simulink model "G2VHDV4"  (R2018b)
settings: Solver=VariableStepAuto  StartTime=0.0  StopTime=1  RelTol=1e-3
undefined symbols (not defined in the file): Ion, Lithium
libraries: powerlib x20, electricdrivelib x1, powerlib_meascontrol x1
settings Model: Creator=user  LastModifiedBy=utkar

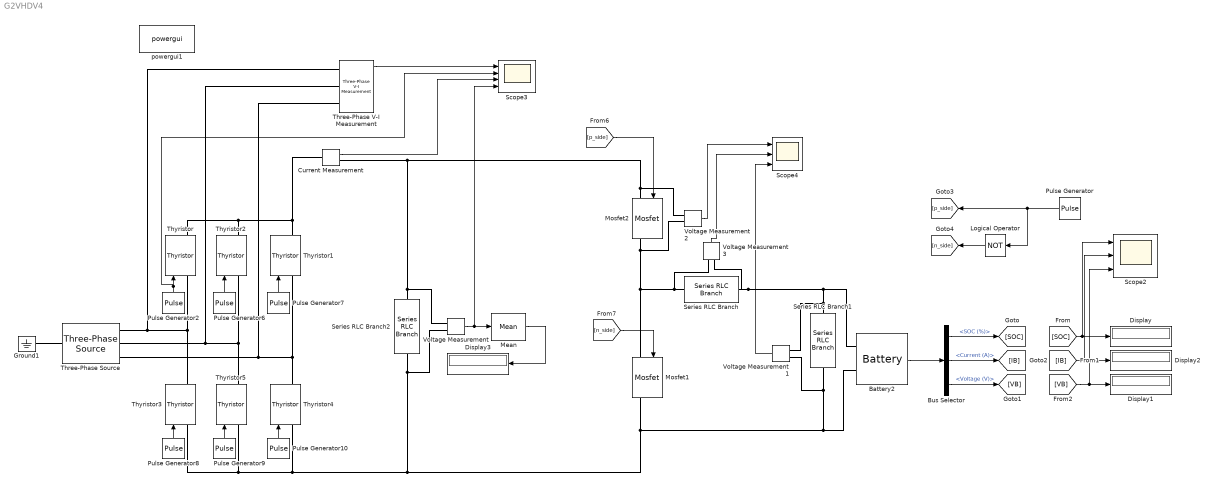
== system G2VHDV4 ==
  Battery2 : electricdrivelib/Extra Sources/Battery  BatType=Lithium-Ion  ShowTempParam=off  ThermalPreset=no  ShowAgeParam=off  NomV=24  NomQ=10  SOC=50  Batt_Tr=1e-4  PresetModel=on  MaxQ=10  MinV=18  FullV=27.9357  Dis_rate=4.3478  R=0.024  Normal_OP=9.0435  expZone="[25.9293     0.491304]"  current=[6.5 13 32.5]  Units=Time  Tci=20  NomT=20  T2=-30  MaxQ2=4.8  FullV2=7.1  Normal_OP2=5.655  expZone2="[6.58           1]"  Rca=0.6  ti=2000  Dp=0  Neq0=0  Tsim=1e6  Ta1=25  Qeol=5.4*0.9  Reol=0.013333*1.2  Char_age=[2.3478, 3]  Dis_age=[2.3478, 10]  N1=1500  N2=10500  N3=1000  N4=1400  Ta2=45  N5=950
  Bus Selector : BusSelector  OutputSignals=SOC (%),Current (A),Voltage (V)
  Current Measurement : powerlib/Measurements/Current Measurement  PhasorSimulation=off  OutputType=Complex  PSBequivalent=0
  Display{,1..3} (4 alike) : Display
  Ground1 : powerlib/Elements/Ground  LConnTagsString=a
  Logical Operator : Logic  Operator=NOT  AllPortsSameDT=off  OutDataTypeStr=boolean
  Mean : powerlib_meascontrol/Measurements/Mean  Freq=50  Vinit=0  Ts=0
  Mosfet1 : powerlib/Power Electronics/Mosfet  Ron=0.1  Lon=0  Rd=0.01  Vfd=0  IC=0  Rs=1e5  Cs=inf  Measurements=on
  Mosfet2 : powerlib/Power Electronics/Mosfet  Ron=0.1  Lon=0  Rd=0.01  Vfd=0  IC=0  Rs=1e5  Cs=inf  Measurements=on
  Pulse Generator : DiscretePulseGenerator  PulseType=Time based  Period=1e-4  PulseWidth=70
  Pulse Generator10 : DiscretePulseGenerator  PulseType=Time based  Period=0.02  PulseWidth=10  PhaseDelay=(1.667e-3)*3+(5.388e-3)
  Pulse Generator2 : DiscretePulseGenerator  PulseType=Time based  Period=0.02  PulseWidth=10  PhaseDelay=(1.667e-3)+(5.388e-3)
  Pulse Generator6 : DiscretePulseGenerator  PulseType=Time based  Period=0.02  PulseWidth=10  PhaseDelay=(1.667e-3)*5+(5.388e-3)
  Pulse Generator7 : DiscretePulseGenerator  PulseType=Time based  Period=0.02  PulseWidth=10  PhaseDelay=(1.667e-3)*9+(5.388e-3)
  Pulse Generator8 : DiscretePulseGenerator  PulseType=Time based  Period=0.02  PulseWidth=10  PhaseDelay=(1.667e-3)*7+(5.388e-3)
  Pulse Generator9 : DiscretePulseGenerator  PulseType=Time based  Period=0.02  PulseWidth=10  PhaseDelay=(1.667e-3)*11+(5.388e-3)
  Scope2 : Scope  NumInputPorts=3
  Scope3 : Scope  NumInputPorts=4
  Scope4 : Scope  NumInputPorts=3
  Series RLC Branch : powerlib/Elements/Series RLC Branch  LConnTagsString=__new0  RConnTagsString=__new0  BranchType=RL  Resistance=0.1  Inductance=1e-3  SetiL0=off  InitialCurrent=0  Capacitance=1e-6  Setx0=off  InitialVoltage=0  Measurements=None
  Series RLC Branch1 : powerlib/Elements/Series RLC Branch  LConnTagsString=__new0  RConnTagsString=__new0  BranchType=RC  Resistance=0.001  Inductance=1e-3  SetiL0=off  InitialCurrent=0  Capacitance=1000e-6  Setx0=off  InitialVoltage=0  Measurements=None
  Series RLC Branch2 : powerlib/Elements/Series RLC Branch  LConnTagsString=__new0  RConnTagsString=__new0  BranchType=R  Resistance=10  Inductance=30e-3  SetiL0=off  InitialCurrent=0  Capacitance=1e-6  Setx0=off  InitialVoltage=0  Measurements=None
  Three-Phase V-I Measurement : powerlib/Measurements/Three-Phase V-I Measurement  VoltageMeasurement=phase-to-ground  SetLabelV=off  LabelV=Vabc  Vpu=off  VpuLL=off  CurrentMeasurement=no  SetLabelI=off  LabelI=Iabc  Ipu=off  Pbase=100e6  Vbase=500e3  OutputType=Complex  PhasorSimulation=off  PSBequivalent=0
  Three-Phase Source : powerlib/Electrical Sources/Three-Phase Source  InternalConnection=Yn  VoltagePhases=off  Voltage=398  PhaseAngle=0  Voltage_phases=[25e3 25e3 25e3]/sqrt(3)  PhaseAngles_phases=[0 -120 +120]  Frequency=50  NonIdealSource=on  SpecifyImpedance=off  Resistance=0  Inductance=0  ShortCircuitLevel=100e6  BaseVoltage=0  XRratio=7  BusType=swing  Pref=10e3  Qref=0  Prefabc=[10e3, 10e3, 10e3]  Qrefabc=[0, 0, 0]  Qmin=-inf  Qmax=inf
  Thyristor{,1..5} (6 alike) : powerlib/Power Electronics/Thyristor  Ron=0  Lon=0  Vf=0  IC=0  Rs=0  Cs=0  Measurements=on
  Voltage Measurement{,1..3} (4 alike) : powerlib/Measurements/Voltage Measurement  PhasorSimulation=off  OutputType=Complex  PSBequivalent=0
  powergui1 : powerlib/powergui  Priority=1  SimulationMode=Continuous  SampleTime=50e-6  frequency=60  Iterations=50  frequencyindice=50  Pbase=100e6  ErrMax=1e-4  UnitsV=kV  UnitsW=MW  buscounter=0  FunctionMessages=off  echomessages=off  EnableUseOfTLC=off  CurrentSourceSwitches=off  DisableSnubberDevices=off  DisableRonSwitches=off  DisableVfSwitches=off  DisplayEquations=off  SolverType=Tustin/Backward Euler (TBE)  Interpol=off  ExternalGateDelay=off  methode=off  Ts=100  x0status=zero  SPID=on  SwTol=0  HookPort=off  RestoreLinks=warning  ResistiveCurrentMeasurement=off  Frange=[0:2:500]  Ylog=off  Xlog=on  ShowGrid=off  save=off  variable=ZData  structure=0  ZoomFFT=off  StartTime=0.0  cycles=1  DisplayStyle=1  fundamental=60  FreqAxis=off  MaxFrequency=1000  frequencyindicesteady=1  RmsSteady=1  display=off
  wires:
  [p_side] -> Mosfet2/1
  Voltage Measurement3/1 -> Scope4/2
  Pulse Generator/1 -> Logical Operator/1, [p_side]
  [SOC] -> Scope2/1, Display/1
  Logical Operator/1 -> [n_side]
  Bus Selector/3 -> [VB]  "<Voltage (V)>"
  [n_side] -> Mosfet1/1
  Voltage Measurement1/1 -> Scope4/3
  Voltage Measurement2/1 -> Scope4/1
  Battery2/1 -> Bus Selector/1
  [VB] -> Scope2/3, Display1/1
  Bus Selector/2 -> [IB]  "<Current (A)>"
  [IB] -> Scope2/2, Display2/1
  Bus Selector/1 -> [SOC]  "<SOC (%)>"
  Pulse Generator8/1 -> Thyristor3/1
  Three-Phase V-I Measurement/1 -> Scope3/1
  Pulse Generator7/1 -> Thyristor1/1
  Pulse Generator6/1 -> Thyristor2/1
  Pulse Generator10/1 -> Thyristor4/1
  Pulse Generator9/1 -> Thyristor5/1
  Voltage Measurement/1 -> Mean/1, Scope3/4
  Pulse Generator2/1 -> Scope3/2, Thyristor/1
  Mean/1 -> Display3/1
  Current Measurement/1 -> Scope3/3
  connections:
  Series RLC Branch1/LConn1 -- Voltage Measurement1/LConn1 -- Series RLC Branch/RConn1 -- Voltage Measurement3/LConn2 -- Battery2/LConn1
  Series RLC Branch/LConn1 -- Voltage Measurement3/LConn1 -- Voltage Measurement2/LConn2 -- Mosfet2/RConn1 -- Mosfet1/LConn1
  Thyristor1/LConn1 -- Three-Phase Source/RConn3 -- Three-Phase V-I Measurement/LConn3 -- Thyristor4/RConn1
  Voltage Measurement1/LConn2 -- Series RLC Branch1/RConn1 -- Battery2/LConn2 -- Mosfet1/RConn1 -- Series RLC Branch2/RConn1 -- Voltage Measurement/LConn2 -- Thyristor4/LConn1 -- Thyristor5/LConn1 -- Thyristor3/LConn1
  Thyristor2/LConn1 -- Thyristor5/RConn1 -- Three-Phase Source/RConn2 -- Three-Phase V-I Measurement/LConn2
  Current Measurement/LConn1 -- Thyristor1/RConn1 -- Thyristor/RConn1 -- Thyristor2/RConn1
  Mosfet2/LConn1 -- Voltage Measurement2/LConn1 -- Series RLC Branch2/LConn1 -- Voltage Measurement/LConn1 -- Current Measurement/RConn1
  Thyristor/LConn1 -- Three-Phase Source/RConn1 -- Three-Phase V-I Measurement/LConn1 -- Thyristor3/RConn1
  Three-Phase Source/LConn1 -- Ground1/LConn1
